simulink model "SG__MDL_DMA_temp"  (R2022b)
settings: Solver=FixedStepAuto  StartTime=0.0  StopTime=Inf  RelTol=1e-3  EnableMultiTasking=on
model workspace (MAT data in the model file):
  N_trig = Simulink.Parameter
  N_trig.Value = 4
  N_trig.Description = 'number of samples for triggered pulse for recording'
  N_trig.DataType = 'auto'
  N_trig.Complexity = 'real'
  N_trig.Dimensions = [1 1]
  dtf_a = Simulink.Parameter
  dtf_a.Value = [1  1  1; 1  1  1; 1  1  1; 1  1  1; 1  1  1; 1  1  1; 1  1  1; 1  1  1; 1  1  1; 1  1  1; 1  1  1; 1  1  1; 1  1  1; 1  1  1; 1  1  1; 1  1  1]
  dtf_a.DataType = 'auto'
  dtf_a.Complexity = 'real'
  dtf_a.Dimensions = [16 3]
  dtf_b = Simulink.Parameter
  dtf_b.Value = [0.5  0.5  0.5; 0.5  0.5  0.5; 0.5  0.5  0.5; 0.5  0.5  0.5; 0.5  0.5  0.5; 0.5  0.5  0.5; 0.5  0.5  0.5; 0.5  0.5  0.5; 0.5  0.5  0.5; 0.5  0.5  0.5; 0.5  0.5  0.5; 0.5  0.5  0.5; 0.5  0.5  0.5; 0.5  0.5  0.5; 0.5  0.5  0.5; 0.5  0.5  0.5]
  dtf_b.DataType = 'auto'
  dtf_b.Complexity = 'real'
  dtf_b.Dimensions = [16 3]
  enable_source = Simulink.Parameter
  enable_source.Value = 1
  enable_source.DataType = 'boolean'
  enable_source.Complexity = 'real'
  enable_source.Dimensions = [1 1]
  freq_fin = Simulink.Parameter
  freq_fin.Value = 1200
  freq_fin.DataType = 'auto'
  freq_fin.Complexity = 'real'
  freq_fin.Dimensions = [1 1]
  freq_ini = Simulink.Parameter
  freq_ini.Value = 150
  freq_ini.DataType = 'auto'
  freq_ini.Complexity = 'real'
  freq_ini.Dimensions = [1 1]
  i2u = Simulink.Parameter
  i2u.Value = 100
  i2u.DataType = 'auto'
  i2u.Complexity = 'real'
  i2u.Dimensions = [1 1]
  k_L = Simulink.Parameter
  k_L.Value = [0; 0; 0; 0; 0; 0; 0; 0; 0; 0; 0; 0; 0; 0; 0; 0]
  k_L.Description = 'Coupling on left of ER. [Linear, NL]'
  k_L.DataType = 'auto'
  k_L.Complexity = 'real'
  k_L.Dimensions = [16 1]
  k_L_NL = Simulink.Parameter
  k_L_NL.Value = [0; 0; 0; 0; 0; 0; 0; 0; 0; 0; 0; 0; 0; 0; 0; 0]
  k_L_NL.Description = 'Coupling on left of ER. [Linear, NL]'
  k_L_NL.DataType = 'auto'
  k_L_NL.Complexity = 'real'
  k_L_NL.Dimensions = [16 1]
  k_O_NL = Simulink.Parameter
  k_O_NL.Value = [0; 0; 0; 0; 0; 0; 0; 0; 0; 0; 0; 0; 0; 0; 0; 0]
  k_O_NL.Description = 'Onsite nonlinearity'
  k_O_NL.DataType = 'auto'
  k_O_NL.Complexity = 'real'
  k_O_NL.Dimensions = [16 1]
  k_R = Simulink.Parameter
  k_R.Value = [0; 0; 0; 0; 0; 0; 0; 0; 0; 0; 0; 0; 0; 0; 0; 0]
  k_R.Description = 'Coupling on right of ER. [Linear, NL]'
  k_R.DataType = 'auto'
  k_R.Complexity = 'real'
  k_R.Dimensions = [16 1]
  k_R_NL = Simulink.Parameter
  k_R_NL.Value = [0; 0; 0; 0; 0; 0; 0; 0; 0; 0; 0; 0; 0; 0; 0; 0]
  k_R_NL.Description = 'Coupling on right of ER. [Linear, NL]'
  k_R_NL.DataType = 'auto'
  k_R_NL.Complexity = 'real'
  k_R_NL.Dimensions = [16 1]
  pb2disp = Simulink.Parameter
  pb2disp.Value = [0; 0; 0; 0; 0; 0; 0; 0; 0; 0; 0; 0; 0; 0; 0; 0]
  pb2disp.DataType = 'auto'
  pb2disp.Complexity = 'real'
  pb2disp.Dimensions = [16 1]
  rec = Simulink.Parameter
  rec.Value = 0
  rec.DataType = 'boolean'
  rec.Complexity = 'real'
  rec.Dimensions = [1 1]
  sens_p = Simulink.Parameter
  sens_p.Value = [0; 0; 0; 0; 0; 0; 0; 0; 0; 0; 0; 0; 0; 0; 0; 0]
  sens_p.DataType = 'auto'
  sens_p.Complexity = 'real'
  sens_p.Dimensions = [16 1]
  src_select = Simulink.Parameter
  src_select.Value = 0
  src_select.DataType = 'auto'
  src_select.Complexity = 'real'
  src_select.Dimensions = [1 1]
  sweep_gain = Simulink.Parameter
  sweep_gain.Value = 0.02
  sweep_gain.DataType = 'auto'
  sweep_gain.Complexity = 'real'
  sweep_gain.Dimensions = [1 1]
  tmax = Simulink.Parameter
  tmax.Value = 2
  tmax.DataType = 'auto'
  tmax.Complexity = 'real'
  tmax.Dimensions = [1 1]
undefined symbols (not defined in the file or in its folder): Ended, Single
libraries: simulink x5, dspsigops x3, speedgoatlib_IO135 x3, speedgoatlib_IO104 x3, hdlsllib x2, dspsrcs4 x2, slrealtimeloglib x1, speedgoatlib_interrupt x1, slrealtimetgmanagement x1, dspsigattribs x1
settings Model: SimulationMode=external  ParamWorkspaceSource=ReferencedWorkspace  DataflowThreadingImplementation=Pthreads  Creator=padlewsk  LastModifiedBy=padlewsk
settings SolverCC: ConcurrentTasks=on  AlgebraicLoopSolver=TrustRegion  PositivePriorityOrder=on  AutoInsertRateTranBlk=on
settings DataIOCC: SaveFormat=StructureWithTime
settings OptimizationCC: DefaultParameterBehavior=Inlined  GainParamInheritBuiltInType=on  UseFloatMulNetSlope=on  InlineInvariantSignals=on  RollThreshold=9  EfficientFloat2IntCast=on  SimCompilerOptimization=on
settings DebuggingCC: TasksWithSamePriorityMsg=none  UnconnectedInputMsg=warning  UnconnectedOutputMsg=warning  UnconnectedLineMsg=warning  ModelReferenceSymbolNameMessage=none
settings HardwareCC: ProdBitPerLong=64  ProdLongLongMode=on  ProdHWDeviceType=Intel->x86-64 (Linux 64)
settings ModelReferenceCC: EnableRefExpFcnMdlSchedulingChecks=on
settings RTWCC: Description=Simulink Real-Time  SystemTargetFile=slrealtime.tlc  TemplateMakefile=slrealtime_default_tmf  Toolchain=Simulink Real-Time Toolchain  BuildConfiguration=Faster Runs  CodeExecutionProfiling=on  TargetLang=C++
settings SimulinkRealTimeTargetCC: UseGCCFastMath=on

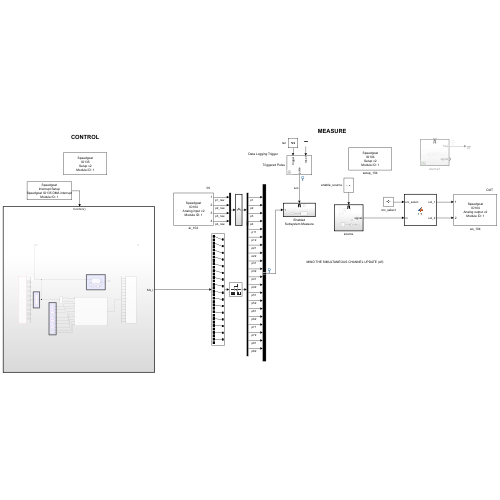
[thumbnail: Simulink's stored preview of the top-level diagram]
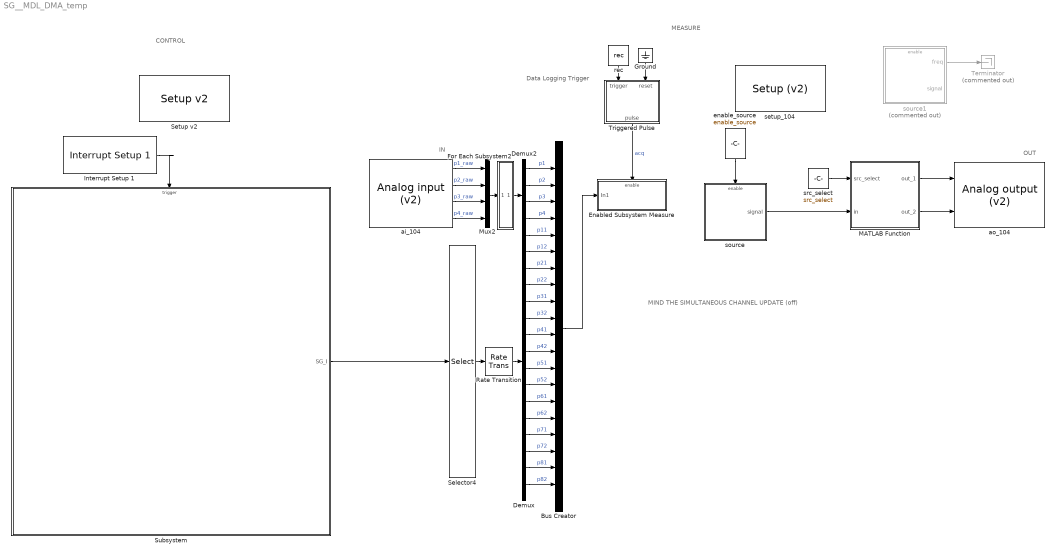
== system SG__MDL_DMA_temp ==
  note: MIND THE SIMULTANEOUS CHANNEL UPDATE (off)
  note: CONTROL
  note: IN
  note: OUT
  note: MEASURE
  note: Data Logging Trigger
  Bus Creator : BusCreator  Inputs=20
  Demux : Demux  Outputs=16
  Demux2 : Demux
  Enabled Subsystem Measure : Subsystem  TreatAsAtomicUnit=on
  For Each Subsystem2 : Subsystem  TreatAsAtomicUnit=on
  Ground : Ground
  Interrupt Setup 1 : speedgoatlib_interrupt/Interrupt Setup 1  parModuleTrigger=off  parPollingMode=off  parPriorityConf=High  parPriority=254  confStartFcn=IO135_start_public  confStopFcn=IO135_stop_public  confIsrFcn=IO135_isr_public  confMapFcn=IO135_map_public  confHookFile=io135_int_hooks.c  confIrqNr=-1  confIsMdlTrig=off  confIsPolling=off  confPriority=254  confModID=16776961  confSelectedInt=Speedgoat IO135 DMA interrupt  confSelectedId=1  confSelectedChannel=[]
  MATLAB Function : MATLAB Function  TreatAsAtomicUnit=on
  Mux2 : Mux
  Rate Transition : RateTransition  Deterministic=off  OutPortSampleTime=0.0001
  Selector4 : Selector  InputPortWidth=32  IndexOptions=Index vector (dialog)  Indices=[1:2:32]  OutputSizes=1
  "Setup v2 " : speedgoatlib_IO135/Setup v2   parPciSlot=-1  parModuleId=1  parInterModuleSync=None  parConvClockBaseRate=60MHz  parConvClock1Divider=2400  parConvClock2Divider=2400  parFrameTriggerEnable=off  parFrameTriggerDivider=10  parConvClock1BaseRate=3  parConvClock2BaseRate=3  parFrameTriggerClock=1  parAdcChannels=[1:32]  parAdcRange1=+-5V  parAdcRange2=+-5V  parAdcRange3=+-5V  parAdcRange4=+-5V  parAdcVoltageRange=[1 1 1 1]  parAdcOversampling1=None  parAdcOversampling2=None  parAdcOversampling3=None  parAdcOversampling4=None  parAdcOversamplRate=[1 1 1 1]  parAdcAutoCorrection=on  parAdcContSampling=off  parAdcDmaEnable=on  parAdcDmaClock=Clock 1  parAdcFrameSize_=1  parAdcSampleTime_=-1  parAdcActiveDmaDevices=[1 1 1 1]  parAdcFrameTriggerEnable=0  parAdcFrameSize=1  parAdcSampleTime=4e-05  parDacChannels=[1:16]  parDacInitValues=0  parDacReset=1  parDacRange1=+-10V  parDacRange2=+-10V  parDacRange3=+-10V  parDacRange4=+-10V  parDacRange5=+-10V  parDacRange6=+-10V  parDacRange7=+-10V  parDacRange8=+-10V  parDacRange9=+-10V  parDacRange10=+-10V  parDacRange11=+-10V  parDacRange12=+-10V  parDacRange13=+-10V  parDacRange14=+-10V  parDacRange15=+-10V  parDacRange16=+-10V  parDacVoltageRange=[5 5 5 5 5 5 5 5 5 5 5 5 5 5 5 5]  parDacAutoCorrection=on  parDacSyncOut=on  parDacDmaEnable=on  parDacDmaLatency=As small as possible  parDacDmaClock=Clock 1  parDacFrameSize_=1  parDacSampleTime_=-1  parDacActiveDmaDevices=[1 1 1 1]  parDacFrameTriggerEnable=0  parDacFrameSize=1  parDacSampleTime=4e-05  parDoChannels=[]  parDoInitValues=0  parDoReset=1  parDiChannels=[]  parDiDebounceEnable=off  parDiDebounceTime=0  parDiDebounceValue=0  parDioPullRefFront=Pull-up 3.3V  parDioPullRefRear=Floating
      settings: SourceProductName=Simulink Real-Time: Speedgoat I/O Blockset
  Subsystem : Subsystem
  Terminator : Terminator  Commented=on
  Triggered Pulse : Subsystem  mask(Triggered Pulse){N=N_trig}
      mask prompts: N "Length (N samples)"
      mask help: Generates a single pulse of N samples length
  ai_104 : speedgoatlib_IO104/Analog input (v2)   parModuleId=1  parTs=0.0001  parPciSlot=-1  parAdChannels=[1,2,3,4]  parAdChannelsSorted=[1,2,3,4]  parAdRange1=+-2.5V  parAdRange2=+-2.5V  parAdCoupling=Single-Ended  parAdFrameSize=1  parAdUseTrigger=off  parAdClockInitiator=Initiator  parAdSampleTime=9.920634921e-07  parTriggerInitiator=Initiator  parTriggerRate=4.161015625e-01
      settings: SourceProductName=Simulink Real-Time: Speedgoat I/O Blockset
  ao_104 : speedgoatlib_IO104/Analog output (v2)   parModuleId=1  parTs=0.0001  parPciSlot=-1  parDaSimultaneous=on  parDaChannels=[1,2]  parDaChannelsSorted=[1,2]  parDaInitValue=[0,0]  parDaReset=[1,1]  parDaRange=+-10V  parDaFrameSize=1  parDaUseTrigger=off  parDaClockInitiator=Initiator  parDaSampleTime=9.920634921e-07  parTriggerInitiator=Initiator  parTriggerRate=4.161015625e-01  parAdBlockPresent=1
      settings: SourceProductName=Simulink Real-Time: Speedgoat I/O Blockset
  enable_source : Constant  Value=enable_source  SampleTime=-1
  rec : Constant  Value=rec  SampleTime=-1
  setup_104 : speedgoatlib_IO104/Setup (v2)   parPciSlot=-1  parModuleId=1  parTriggerInitiator=Initiator  parTriggerRate=4.161015625e-01  parCalibrate=off  parAdChannels=[1:4]  parAdRange1=+-2.5V  parAdRange2=+-2.5V  parAdCoupling=Single-Ended  parAdUseTrigger=off  parAdFrameSize=1  parAdClockInitiator=Initiator  parAdSampleTime=9.920634921e-07  parDaSimultaneous=on  parDaChannels=[1:2]  parDaChannelsSorted=[1,2]  parDaInitValue=[0]  parDaReset=[1]  parDaRange=+-10V  parDaUseTrigger=off  parDaFrameSize=1  parDaClockInitiator=Initiator  parDaSampleTime=9.920634921e-07  parDioByte0Dir=Outputs  parDioByte1Dir=Inputs  parDoChannels=[]  parDoInitValues=[0]  parDoReset=[1]  parDiChannels=[]
      settings: SourceProductName=Simulink Real-Time: Speedgoat I/O Blockset
  source : Subsystem  TreatAsAtomicUnit=on
  source1 : Subsystem  Commented=on  TreatAsAtomicUnit=on
  src_select : Constant  Value=src_select
  wires:
  enable_source/1 -> source/Enable
  Triggered Pulse/1(pulse) -> Enabled Subsystem Measure/Enable  "acq"
  Ground/1 -> Triggered Pulse/2(reset)
  rec/1 -> Triggered Pulse/1(trigger)
  Bus Creator/1 -> Enabled Subsystem Measure/1(In1)
  source1/1(freq) -> Terminator/1
  source/1(signal) -> MATLAB Function/2(in)
  src_select/1 -> MATLAB Function/1(src_select)
  MATLAB Function/1(out_1) -> ao_104/1
  MATLAB Function/2(out_2) -> ao_104/2
  For Each Subsystem2/1(Out1) -> Demux2/1
  Mux2/1 -> For Each Subsystem2/1(In1)
  ai_104/1 -> Mux2/1  "p1_raw"
  ai_104/2 -> Mux2/2  "p2_raw"
  ai_104/3 -> Mux2/3  "p3_raw"
  ai_104/4 -> Mux2/4  "p4_raw"
  Demux2/2 -> Bus Creator/2  "p2"
  Demux2/1 -> Bus Creator/1  "p1"
  Demux2/3 -> Bus Creator/3  "p3"
  Demux2/4 -> Bus Creator/4  "p4"
  Demux/1 -> Bus Creator/5  "p11"
  Demux/2 -> Bus Creator/6  "p12"
  Demux/3 -> Bus Creator/7  "p21"
  Demux/4 -> Bus Creator/8  "p22"
  Demux/5 -> Bus Creator/9  "p31"
  Demux/6 -> Bus Creator/10  "p32"
  Demux/7 -> Bus Creator/11  "p41"
  Demux/8 -> Bus Creator/12  "p42"
  Demux/9 -> Bus Creator/13  "p51"
  Demux/10 -> Bus Creator/14  "p52"
  Demux/11 -> Bus Creator/15  "p61"
  Demux/12 -> Bus Creator/16  "p62"
  Demux/13 -> Bus Creator/17  "p71"
  Demux/14 -> Bus Creator/18  "p72"
  Demux/15 -> Bus Creator/19  "p81"
  Demux/16 -> Bus Creator/20  "p82"
  Selector4/1 -> Rate Transition/1
  Rate Transition/1 -> Demux/1
  Subsystem/1(SG_I) -> Selector4/1
  Interrupt Setup 1/1 -> Subsystem/Trigger

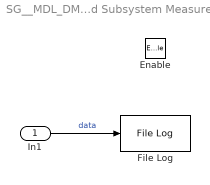
== system SG__MDL_DMA_temp/Enabled Subsystem Measure ==
  In1 : Inport
  Enable : EnablePort
  File Log : slrealtimeloglib/File Log  decimation=1  inputProcessing=Elements as channels (sample based)
  wires:
  In1/1 -> File Log/1  "data"

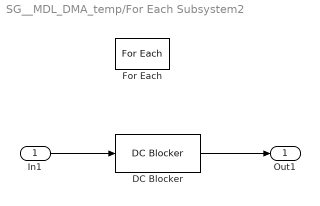
== system SG__MDL_DMA_temp/For Each Subsystem2 ==
  In1 : Inport  Partition=on  PartitionDimension=1  PartitionWidth=1  PartitionOffset=0
  DC Blocker : dspsigops/DC Blocker  Algorithm=FIR  NormalizedBandwidth=0.001  Length=50  Order=6  SimulateUsing=Code generation
      settings: LibrarySourceBlock=dsphdlsupportsigops/DC Blocker
  For Each : ForEach  DisableCoverage=on
  Out1 : Outport  ConcatenationDimension=1
  wires:
  In1/1 -> DC Blocker/1
  DC Blocker/1 -> Out1/1

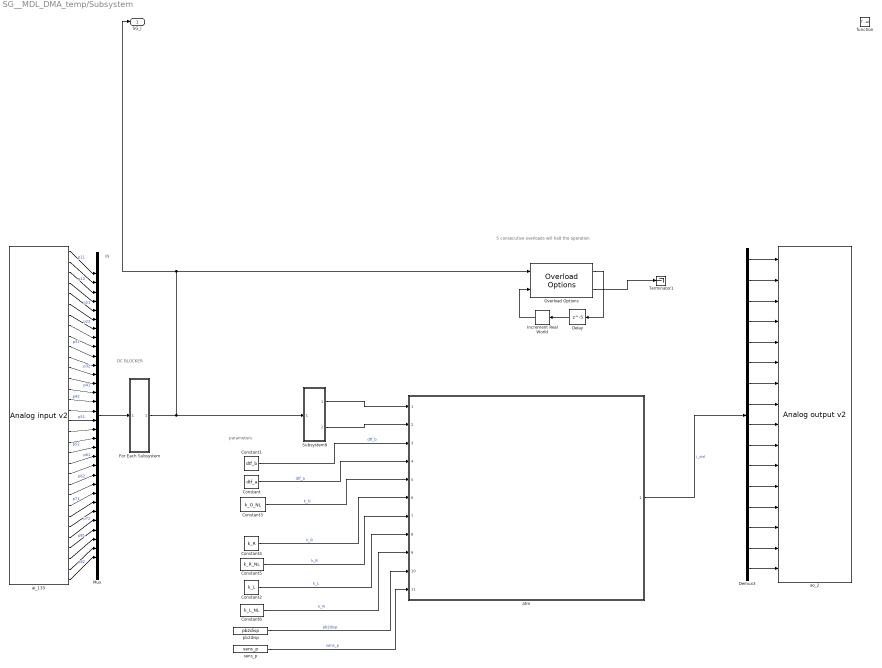
== system SG__MDL_DMA_temp/Subsystem ==
  note: DC BLOCKER
  note: 5 consecutive overloads will halt the operation
  note: IN
  note: parameters
  function : TriggerPort  TriggerType=function-call  VariantControl=(inherit)
  Constant : Constant  Value=dtf_a  SampleTime=-1
  Constant1 : Constant  Value=dtf_b  SampleTime=-1
  Constant2 : Constant  Value=k_L  SampleTime=-1
  Constant3 : Constant  Value=k_O_NL  SampleTime=-1
  Constant4 : Constant  Value=k_R  SampleTime=-1
  Constant5 : Constant  Value=k_R_NL  SampleTime=-1
  Constant6 : Constant  Value=k_L_NL  SampleTime=-1
  Delay : Delay  DelayLength=5
  Demux3 : Demux  Outputs=16
  For Each Subsystem : Subsystem  TreatAsAtomicUnit=on
  Increment Real World : simulink/Additional Math & Discrete/Additional Math: Increment - Decrement/Increment Real World
  Mux : Mux  Inputs=32
  Overload Options : slrealtimetgmanagement/Overload Options  startupDur=1  startupDurSrc=Tunable Parameter  maxOverload=0  maxOverloadSrc=Input Port  TETFlag=on
  Subsystem8 : Subsystem
  Terminator1 : Terminator
  ai_135 : speedgoatlib_IO135/Analog input v2   parModuleId=1  parSampleTime=-1  parPciSlot=-1  parAdcChannels=[1 2 3 4 5 6 7 8 9 10 11 12 13 14 15 16 17 18 19 20 21 22 23 24 25 26 27 28 29 30 31 32]  parAdcVoltageRange=[1 1 1 1]  parAdcOversamplRate=[1 1 1 1]  parAdcContSampling=0  parAdcDmaEnable=1  parAdcActiveDmaDevices=[1 1 1 1]  parAdcFrameSize=1
      settings: SourceProductName=Simulink Real-Time: Speedgoat I/O Blockset
  ao_2 : speedgoatlib_IO135/Analog output v2   parModuleId=1  parSampleTime=-1  parPciSlot=-1  parDacChannels=[1 2 3 4 5 6 7 8 9 10 11 12 13 14 15 16]  parDacVoltageRange=[5 5 5 5 5 5 5 5 5 5 5 5 5 5 5 5]  parDacInitValues=[0 0 0 0 0 0 0 0 0 0 0 0 0 0 0 0]  parDacReset=[1 1 1 1 1 1 1 1 1 1 1 1 1 1 1 1]  parDacSyncOut=1  parDacDmaEnable=1  parDacActiveDmaDevices=[1 1 1 1]  parDacDmaLatency=1  parDacFrameSize=1
      settings: SourceProductName=Simulink Real-Time: Speedgoat I/O Blockset
  atm : Subsystem  ReferencedSubsystem=atm
  pb2disp : Constant  Value=pb2disp  SampleTime=-1
  sens_p : Constant  Value=sens_p  SampleTime=-1
  SG_I : Outport
  wires:
  ai_135/10 -> Mux/10
  ai_135/17 -> Mux/17  "p51"
  Constant2/1 -> atm/8  "k_L"
  Overload Options/1 -> Delay/1
  ai_135/29 -> Mux/29  "p81"
  ai_135/28 -> Mux/28
  ai_135/26 -> Mux/26
  ai_135/8 -> Mux/8
  ai_135/3 -> Mux/3  "p12"
  Demux3/10 -> ao_2/10
  ai_135/6 -> Mux/6
  ai_135/4 -> Mux/4
  pb2disp/1 -> atm/10  "pb2disp"
  ai_135/9 -> Mux/9  "p31"
  ai_135/21 -> Mux/21  "p61"
  Mux/1 -> For Each Subsystem/1(In1)
  Demux3/5 -> ao_2/5
  Demux3/12 -> ao_2/12
  ai_135/14 -> Mux/14
  Demux3/15 -> ao_2/15
  For Each Subsystem/1(SG_I) -> Subsystem8/1(SG_I), SG_I/1, Overload Options/1
  ai_135/15 -> Mux/15  "p42"
  ai_135/25 -> Mux/25  "p71"
  ai_135/20 -> Mux/20
  ai_135/12 -> Mux/12
  Constant/1 -> atm/4  "dtf_a"
  ai_135/7 -> Mux/7  "p22"
  sens_p/1 -> atm/11  "sens_p"
  ai_135/2 -> Mux/2
  Demux3/9 -> ao_2/9
  ai_135/30 -> Mux/30
  Constant5/1 -> atm/7  "k_R"
  ai_135/5 -> Mux/5  "p21"
  Constant4/1 -> atm/6  "k_R"
  Demux3/14 -> ao_2/14
  ai_135/24 -> Mux/24
  ai_135/19 -> Mux/19  "p52"
  Constant3/1 -> atm/5  "k_O"
  ai_135/23 -> Mux/23  "p62"
  Increment Real World/1 -> Overload Options/2
  Delay/1 -> Increment Real World/1
  Demux3/2 -> ao_2/2
  ai_135/11 -> Mux/11  "p32"
  ai_135/18 -> Mux/18
  Demux3/3 -> ao_2/3
  Demux3/16 -> ao_2/16
  ai_135/27 -> Mux/27  "p72"
  ai_135/13 -> Mux/13  "p41"
  ai_135/32 -> Mux/32
  Demux3/7 -> ao_2/7
  ai_135/31 -> Mux/31  "p82"
  Demux3/13 -> ao_2/13
  Overload Options/2 -> Terminator1/1
  Demux3/4 -> ao_2/4
  Demux3/1 -> ao_2/1
  Demux3/8 -> ao_2/8
  Demux3/11 -> ao_2/11
  Subsystem8/2(Input1) -> atm/2
  ai_135/16 -> Mux/16
  ai_135/1 -> Mux/1  "p11"
  Demux3/6 -> ao_2/6
  Constant6/1 -> atm/9  "k_R"
  ai_135/22 -> Mux/22
  atm/1 -> Demux3/1  "i_ctrl"
  Subsystem8/1(Input) -> atm/1
  Constant1/1 -> atm/3  "dtf_b"

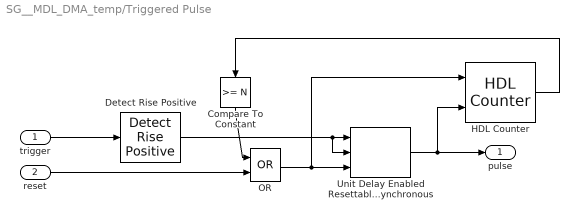
== system SG__MDL_DMA_temp/Triggered Pulse ==
  trigger : Inport
  reset : Inport  Port=2
  Compare To Constant : simulink/Logic and Bit Operations/Compare To Constant  relop=>=  const=N  OutDataTypeStr=boolean
  Detect Rise Positive : simulink/Logic and Bit Operations/Detect Rise Positive  vinit=0  OutDataTypeStr=boolean
  HDL Counter : hdlsllib/Sources/HDL Counter  CountType=Free running  CountInit=1  CountStep=1  CountMax=25  CountFromType=Initial value  CountFrom=1  CountResetPort=on  CountLoadPort=off  CountEnbPort=on  CountDirPort=off  CountHitOutputPort=off  CountDataType=Unsigned  CountWordLen=32  CountFracLen=0  CountSampTime=1
  OR : Logic  Operator=OR  AllPortsSameDT=off  OutDataTypeStr=boolean
  Unit Delay Enabled Resettable Synchronous : hdlsllib/Discrete/Unit Delay Enabled Resettable Synchronous  InitialCondition=0.0  SampleTime=-1
  pulse : Outport  VectorParamsAs1DForOutWhenUnconnected=off
  wires:
  OR/1 -> Unit Delay Enabled Resettable Synchronous/3, HDL Counter/1
  trigger/1 -> Detect Rise Positive/1
  Unit Delay Enabled Resettable Synchronous/1 -> HDL Counter/2, pulse/1
  Compare To Constant/1 -> OR/1
  reset/1 -> OR/2
  Detect Rise Positive/1 -> Unit Delay Enabled Resettable Synchronous/1, Unit Delay Enabled Resettable Synchronous/2
  HDL Counter/1 -> Compare To Constant/1

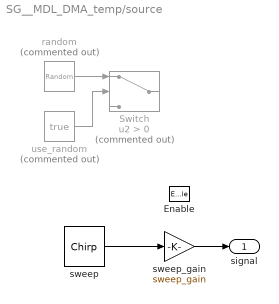
== system SG__MDL_DMA_temp/source ==
  Enable : EnablePort  StatesWhenEnabling=reset
  Switch : Switch  Commented=on  Criteria=u2 > Threshold  SaturateOnIntegerOverflow=off  InputSameDT=off
  random : RandomNumber  Commented=on  Variance=0.5  SampleTime=3.5e-05
  sweep : dspsrcs4/Chirp  sweep=Logarithmic  mode=Bidirectional  f0=freq_ini  f1=freq_fin  t1=tmax  Tsweep=tmax  phase=0  Ts=0.0001  spf=1  datatype=Double  OutputFrames=off
  sweep_gain : Gain  Gain=sweep_gain
  use_random : Constant  Commented=on  Value=true  SampleTime=-1
  signal : Outport  OutputWhenDisabled=reset  InitialOutput=0  VectorParamsAs1DForOutWhenUnconnected=off
  wires:
  use_random/1 -> Switch/2
  random/1 -> Switch/1
  sweep/1 -> sweep_gain/1
  sweep_gain/1 -> signal/1

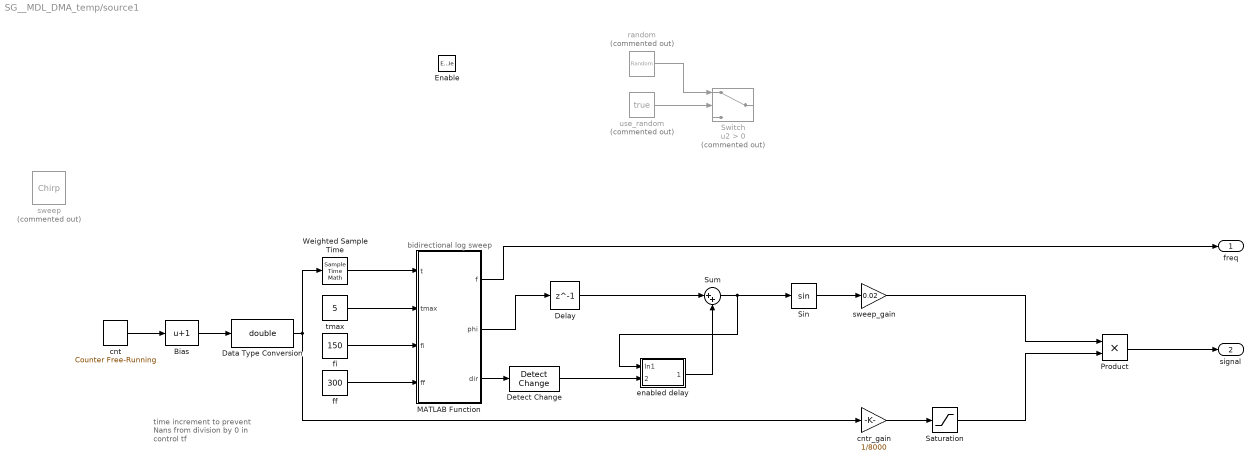
== system SG__MDL_DMA_temp/source1 ==
  note: bidirectional log sweep
  note: time increment to prevent Nans from division by 0 in control tf
  Enable : EnablePort  StatesWhenEnabling=reset
  Bias : Bias  Bias=1  SaturateOnIntegerOverflow=off
  Data Type Conversion : DataTypeConversion  OutDataTypeStr=double  SaturateOnIntegerOverflow=off  RndMeth=Floor
  Delay : Delay  DelayLength=1
  Detect Change : simulink/Logic and Bit Operations/Detect Change  vinit=false  OutDataTypeStr=boolean
  MATLAB Function : MATLAB Function  TreatAsAtomicUnit=on
  Product : Product
  Saturation : Saturate  UpperLimit=1  LowerLimit=0
  Sin : Trigonometry
  Sum : Sum  Inputs=|++
  Switch : Switch  Commented=on  Criteria=u2 > Threshold  SaturateOnIntegerOverflow=off  InputSameDT=off
  Weighted Sample Time : SampleTimeMath  TsampMathOp=*
  cnt : simulink/Sources/Counter Free-Running  NumBits=32  tsamp=-1
  cntr_gain : Gain  Gain=1/8000  ParamDataTypeStr=double
  enabled delay : Subsystem
  ff : Constant  Value=300
  fi : Constant  Value=150
  random : RandomNumber  Commented=on  Variance=0.5  SampleTime=3.5e-05
  sweep : dspsrcs4/Chirp  Commented=on  sweep=Logarithmic  mode=Bidirectional  f0=150  f1=1200  t1=10  Tsweep=20  phase=0  Ts=3.5e-05  spf=1  datatype=Double  OutputFrames=off
  sweep_gain : Gain  Gain=0.02
  tmax : Constant  Value=5
  use_random : Constant  Commented=on  Value=true  SampleTime=-1
  freq : Outport  OutputWhenDisabled=reset  InitialOutput=0  VectorParamsAs1DForOutWhenUnconnected=off
  signal : Outport  Port=2  OutputWhenDisabled=reset  InitialOutput=0  VectorParamsAs1DForOutWhenUnconnected=off
  wires:
  use_random/1 -> Switch/2
  random/1 -> Switch/1
  sweep_gain/1 -> Product/1
  cntr_gain/1 -> Saturation/1
  Product/1 -> signal/1
  MATLAB Function/2(phi) -> Delay/1
  Saturation/1 -> Product/2
  Weighted Sample Time/1 -> MATLAB Function/1(t)
  Data Type Conversion/1 -> cntr_gain/1, Weighted Sample Time/1
  MATLAB Function/1(f) -> freq/1
  Sin/1 -> sweep_gain/1
  MATLAB Function/3(dir) -> Detect Change/1
  Detect Change/1 -> enabled delay/2(enable)
  Delay/1 -> Sum/1
  enabled delay/1(Out1) -> Sum/2
  Sum/1 -> enabled delay/1(In1), Sin/1
  cnt/1 -> Bias/1
  Bias/1 -> Data Type Conversion/1
  ff/1 -> MATLAB Function/4(ff)
  tmax/1 -> MATLAB Function/2(tmax)
  fi/1 -> MATLAB Function/3(fi)

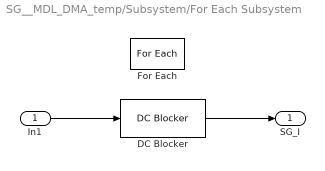
== system SG__MDL_DMA_temp/Subsystem/For Each Subsystem ==
  In1 : Inport  Partition=on  PartitionDimension=1  PartitionWidth=1  PartitionOffset=0
  DC Blocker : dspsigops/DC Blocker  Algorithm=FIR  NormalizedBandwidth=0.001  Length=20  Order=6  SimulateUsing=Code generation
      settings: LibrarySourceBlock=dsphdlsupportsigops/DC Blocker
  For Each : ForEach  DisableCoverage=on
  SG_I : Outport  ConcatenationDimension=1
  wires:
  In1/1 -> DC Blocker/1
  DC Blocker/1 -> SG_I/1

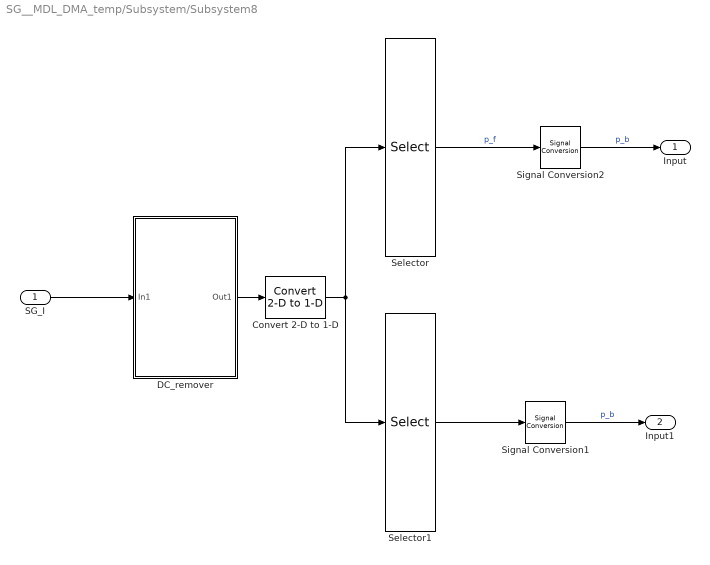
== system SG__MDL_DMA_temp/Subsystem/Subsystem8 ==
  SG_I : Inport
  Convert 2-D to 1-D : dspsigattribs/Convert 2-D to 1-D
  DC_remover : Subsystem  TreatAsAtomicUnit=on
      settings: RTWSystemCode=Nonreusable function
  Selector : Selector  InputPortWidth=32  IndexOptions=Index vector (dialog)  Indices=1:2:32  OutputSizes=1
  Selector1 : Selector  InputPortWidth=32  IndexOptions=Index vector (dialog)  Indices=2:2:32  OutputSizes=1
  Signal Conversion1 : SignalConversion  OverrideOpt=off
  Signal Conversion2 : SignalConversion  OverrideOpt=off
  Input : Outport
  Input1 : Outport  Port=2
  wires:
  SG_I/1 -> DC_remover/1(In1)
  Selector1/1 -> Signal Conversion1/1
  DC_remover/1(Out1) -> Convert 2-D to 1-D/1
  Selector/1 -> Signal Conversion2/1  "p_f"
  Signal Conversion1/1 -> Input1/1  "p_b"
  Signal Conversion2/1 -> Input/1  "p_b"
  Convert 2-D to 1-D/1 -> Selector/1, Selector1/1

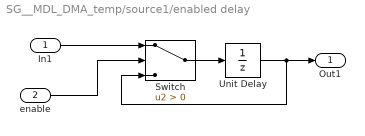
== system SG__MDL_DMA_temp/source1/enabled delay ==
  In1 : Inport
  enable : Inport  Port=2
  Switch : Switch  Criteria=u2 > Threshold  SaturateOnIntegerOverflow=off  InputSameDT=off
  Unit Delay : UnitDelay  SampleTime=-1  HasFrameUpgradeWarning=on
  Out1 : Outport
  wires:
  Unit Delay/1 -> Switch/3, Out1/1
  Switch/1 -> Unit Delay/1
  In1/1 -> Switch/1
  enable/1 -> Switch/2

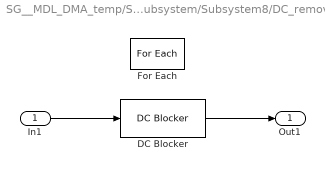
== system SG__MDL_DMA_temp/Subsystem/Subsystem8/DC_remover ==
  In1 : Inport  Partition=on  PartitionDimension=1  PartitionWidth=1  PartitionOffset=0
  DC Blocker : dspsigops/DC Blocker  Algorithm=FIR  NormalizedBandwidth=0.001  Length=20  Order=6  SimulateUsing=Code generation
      settings: LibrarySourceBlock=dsphdlsupportsigops/DC Blocker
  For Each : ForEach  DisableCoverage=on
  Out1 : Outport  ConcatenationDimension=1
  wires:
  In1/1 -> DC Blocker/1
  DC Blocker/1 -> Out1/1

== matlab function SG__MDL_DMA_temp/source1/MATLAB Function ==
  data: f output; t input; tmax input; phi output; dir output; fi input; ff input
function [f, phi, dir] = fcn(t, tmax, fi, ff)
%tmax is the time at which the maximum frequency is reached

t = mod(t, 2*tmax);

if t < tmax
    % up
    dir = 1;
    
    
    % linear (CF wikipedia)
%     phi = 2*pi*(0.5*(ff - fi)*t^2/tmax + fi*t);
%     f = fi + (ff - fi)*t/tmax;
    
    % logarithmic %%% https://en.wikipedia.org/wiki/Chirp
    k = log((ff/fi)^(1/tmax));
    phi = 2*pi*fi*(exp(k*t) - 1)/k;
    f = fi*exp(k*t);
else
    % down
    dir = -1;
    
    
    % linear (CF wikipedia)
%     phi = 2*pi*(0.5*(fi - ff)*(t-tmax)^2/tmax + ff*(t-tmax)); % linear
%     f = ff + (fi - ff)*(t - tmax)/tmax;
    
    % logarithmic
    k = log((fi/ff)^(1/tmax));
    phi = 2*pi*ff*(exp(k*(t - tmax)) - 1)/k;
    f = ff*exp(k*(t-tmax));
end

phi = mod(phi, 2*pi);

== matlab function SG__MDL_DMA_temp/MATLAB Function ==
  data: src_select input; in input; out_1 output; out_2 output
function [out_1, out_2] = fct(src_select, in)
out_1 = 0;
out_2 = 0;
if src_select == 1
    out_1 = in;
elseif src_select == 2
    out_2 = in;
end
